simulink model "SimscapeCrane_StepInput"  (R2015a)
settings: Solver=ode15s  StartTime=0.0  StopTime=T  RelTol=1e-3
values from neighbouring files (symbols this model uses):
  filter_denominator = cell2mat(disc_filter.den)    [test.m]
  filter_numerator = cell2mat(disc_filter.num)    [test.m]
  m = 0.47    [Params_Simscape.mat]
  MR = 1.71    [Params_Simscape.mat]
  Ts_hw = 0.01    [test.m]
  TxBreak = 0    [Params_Simscape.mat]
  TxCoulomb = 3.7489    [Params_Simscape.mat]
  TxVisc = 58.085    [Params_Simscape.mat]
  TyBreak = 0    [Params_Simscape.mat]
  TyCoulomb = 2.674    [Params_Simscape.mat]
  TzBreak = 0    [Params_Simscape.mat]
  TzCoulomb = 6.1    [Params_Simscape.mat]
  xRange = [0 0.52]    [Params_Simscape.mat]
  xZero = 0.3    [Params_Simscape.mat]
  yRange = [0 0.62]    [Params_Simscape.mat]
  yZero = 0.3    [Params_Simscape.mat]
  zRange = [0.17 0.8]    [Params_Simscape.mat]
  zZero = 0.47    [Params_Simscape.mat]
undefined symbols (not defined in the file or in its folder): Ts, X, x_init, Y, Z
undefined symbols (not defined in the file): M, TorqueMultX, TorqueMultY, TorqueMultZ, TxTrans, TyTrans, TyVisc, TzTrans, TzVisc
libraries: sm_lib x146, fl_lib x62, nesl_utility x24, elec_lib x9, simulink x9, sm_double_wishbone_suspension_lib x4, aerolibtransform2 x1
(part 2 of 15)

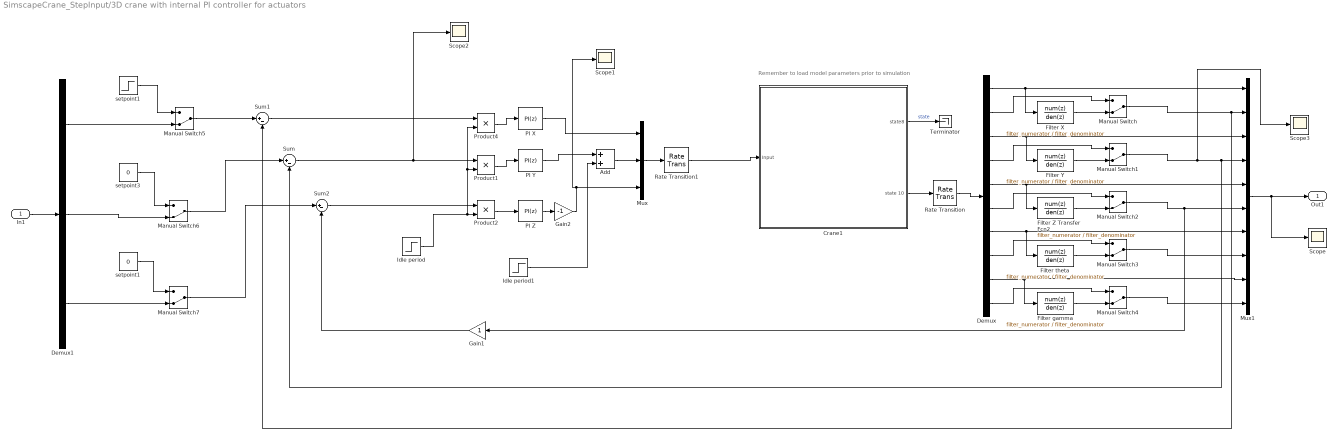
== system SimscapeCrane_StepInput/3D crane with internal PI controller for actuators ==
  note: Remember to load model parameters prior to simulation
  In1 : Inport
  " setpoint1" : Step  Time=1.5  After=-0.05  SampleTime=0
  Add : Sum
  Crane1 : Subsystem  mask{penduMass=m, cartMass=M, MR=MR, xRange=xRange, yRange=yRange, zRange=zRange, xZero=xZero, yZero=yZero, zZero=zZero, TxBreak=TxBreak, TxCoulomb=TxCoulomb, TxVisc=TxVisc, TxTrans=TxTrans, TyBreak=TyBreak, TyCoulomb=TyCoulomb, TyVisc=TyVisc, TyTrans=TyTrans, TzBreak=TzBreak, TzCoulomb=TzCoulomb, TzVisc=TzVisc, TzTrans=TzTrans, Ux=TorqueMultX, Uy=TorqueMultY, Uz=TorqueMultZ}
      mask prompts: penduMass "Pendulum Mass (Kg)"; cartMass "Mass of the cart (Kg)"; MR "Mass of the rail (Kg)"; TxBreak "BreakAwayFriction"; TxCoulomb "Coulomb Friction"; TxVisc "Viscous friction"; TxTrans "Transition coeff"; TyBreak "BreakAwayFriction"; TyCoulomb "Coulomb Friction"; TyVisc "Viscous friction"; TyTrans "Transition coeff"; TzBreak "BreakAwayFriction"; TzCoulomb "Coulomb Friction"; TzVisc "Viscous friction"; TzTrans "Transition coeff"; Ux "Rail motor multiplier (X)"; Uy "Cart motor multiplier (Y)"; Uz "String motor multiplier (Z)"
      mask init:
      | %mass lowSat
      | penduMass=max(penduMass,1e-3);
      | cartMass=max(cartMass,1e-3);
      | MR=max(MR,1e-3);
      | 
      | %zeros saturated
      | xZero=max(xZero,xRange(1));
      | xZero=min(xZero,xRange(2));
      | 
      | yZero=max(yZero,yRange(1));
      | yZero=min(yZero,yRange(2));
      | 
      | zZero=max(zZero,zRange(1));
      | zZero=min(zZero,zRange(2));
      mask DialogControl DescGroupVar Prompt: 3D Crane Simscape model
      mask Display:
